simulink model "Simulator"  (R2016a)
settings: Solver=VariableStepAuto  StartTime=0.0  StopTime=10.0  RelTol=1e-6
undefined symbols (not defined in the file): eta_0, I_g, m, M_A, M_RB, nu_0, r_bg
libraries: SimulatorLibrary x5
settings Model: Creator=MortenFyhn  LastModifiedBy=vegard
settings DataIOCC: LimitDataPoints=on
settings DebuggingCC: AllowSymbolicDim=off
settings ModelReferenceCC: PropagateSignalLabelsOutOfModel=off
settings GRTTargetCC: GeneratePreprocessorConditionals=Use local settings

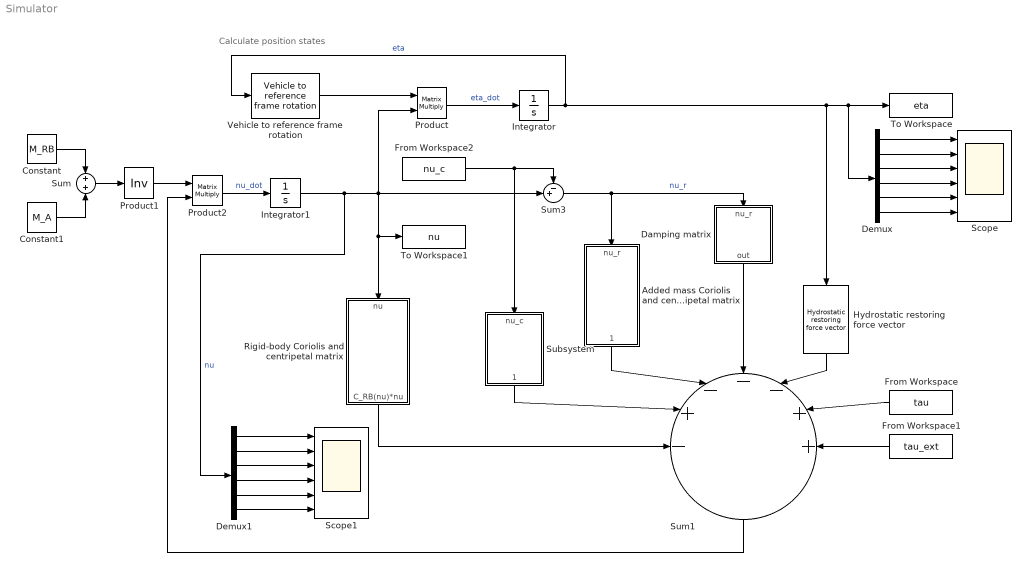
== system Simulator ==
  note: Calculate position states
  Added mass Coriolis and centripetal matrix : Subsystem
  Constant : Constant  Value=M_RB
  Constant1 : Constant  Value=M_A
  Damping matrix : Subsystem
  Demux : Demux  Outputs=6
  Demux1 : Demux  Outputs=6
  From Workspace : FromWorkspace  VariableName=tau  SampleTime=0
  From Workspace1 : FromWorkspace  VariableName=tau_ext  SampleTime=0
  From Workspace2 : FromWorkspace  VariableName=nu_c  SampleTime=0
  Hydrostatic restoring force vector : SimulatorLibrary/Hydrostatic restoring force vector
  Integrator : Integrator  InitialCondition=eta_0
  Integrator1 : Integrator  InitialCondition=nu_0
  Product : Product  Multiplication=Matrix(*)
  Product1 : Product  Inputs=/  Multiplication=Matrix(*)
  Product2 : Product  Multiplication=Matrix(*)
  Rigid-body Coriolis and centripetal matrix : Subsystem
  Scope : Scope  NumInputPorts=6
  Scope1 : Scope  NumInputPorts=6
  Subsystem : Subsystem
  Sum : Sum  Inputs=+|+
  Sum1 : Sum  Inputs=-+---++
  Sum3 : Sum  Inputs=-+|
  To Workspace : ToWorkspace  VariableName=eta  SaveFormat=Timeseries  SampleTime=-1
  To Workspace1 : ToWorkspace  VariableName=nu  SaveFormat=Timeseries  SampleTime=-1
  Vehicle to reference frame rotation : SimulatorLibrary/Vehicle to reference frame rotation
  wires:
  Vehicle to reference frame rotation/1 -> Product/1
  Product/1 -> Integrator/1  "eta_dot"
  Integrator/1 -> Vehicle to reference frame rotation/1, Demux/1, To Workspace/1, Hydrostatic restoring force vector/1  "eta"
  Constant1/1 -> Sum/2
  Constant/1 -> Sum/1
  Sum/1 -> Product1/1
  Product1/1 -> Product2/1
  Product2/1 -> Integrator1/1  "nu_dot"
  Integrator1/1 -> Demux1/1, To Workspace1/1, Rigid-body Coriolis and centripetal matrix/1(nu), Sum3/2, Product/2  "nu"
  Sum3/1 -> Added mass Coriolis and centripetal matrix/1(nu_r), Damping matrix/1(nu_r)  "nu_r"
  Sum1/1 -> Product2/2
  Hydrostatic restoring force vector/1 -> Sum1/5
  From Workspace/1 -> Sum1/6
  From Workspace1/1 -> Sum1/7
  Rigid-body Coriolis and centripetal matrix/1(C_RB(nu)*nu) -> Sum1/1
  Subsystem/1(M_A nu_c_dot) -> Sum1/2
  Added mass Coriolis and centripetal matrix/1(C_A(nu_r) nu_r) -> Sum1/3
  Damping matrix/1(out) -> Sum1/4
  From Workspace2/1 -> Subsystem/1(nu_c), Sum3/1
  Demux/6 -> Scope/6
  Demux/5 -> Scope/5
  Demux/4 -> Scope/4
  Demux/3 -> Scope/3
  Demux/2 -> Scope/2
  Demux/1 -> Scope/1
  Demux1/6 -> Scope1/6
  Demux1/5 -> Scope1/5
  Demux1/4 -> Scope1/4
  Demux1/3 -> Scope1/3
  Demux1/2 -> Scope1/2
  Demux1/1 -> Scope1/1

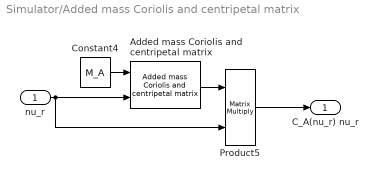
== system Simulator/Added mass Coriolis and centripetal matrix ==
  nu_r : Inport
  Added mass Coriolis and centripetal matrix : SimulatorLibrary/Added mass Coriolis and centripetal matrix
  Constant4 : Constant  Value=M_A
  Product5 : Product  Multiplication=Matrix(*)
  C_A(nu_r) nu_r : Outport
  wires:
  Constant4/1 -> Added mass Coriolis and centripetal matrix/1
  Added mass Coriolis and centripetal matrix/1 -> Product5/1
  nu_r/1 -> Product5/2, Added mass Coriolis and centripetal matrix/2
  Product5/1 -> C_A(nu_r) nu_r/1

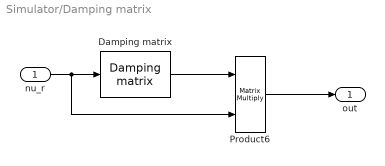
== system Simulator/Damping matrix ==
  nu_r : Inport
  Damping matrix : SimulatorLibrary/Damping matrix
  Product6 : Product  Multiplication=Matrix(*)
  out : Outport
  wires:
  Damping matrix/1 -> Product6/1
  nu_r/1 -> Product6/2, Damping matrix/1
  Product6/1 -> out/1

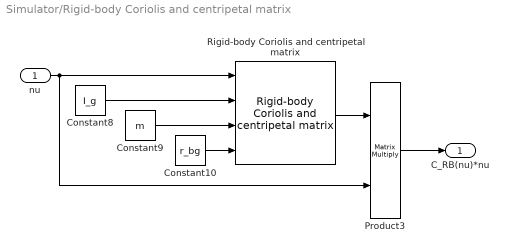
== system Simulator/Rigid-body Coriolis and centripetal matrix ==
  nu : Inport
  Constant10 : Constant  Value=r_bg
  Constant8 : Constant  Value=I_g
  Constant9 : Constant  Value=m
  Product3 : Product  Multiplication=Matrix(*)
  Rigid-body Coriolis and centripetal matrix : SimulatorLibrary/Rigid-body Coriolis and centripetal matrix
  C_RB(nu)*nu : Outport
  wires:
  Constant10/1 -> Rigid-body Coriolis and centripetal matrix/4
  Constant8/1 -> Rigid-body Coriolis and centripetal matrix/2
  Rigid-body Coriolis and centripetal matrix/1 -> Product3/1
  Constant9/1 -> Rigid-body Coriolis and centripetal matrix/3
  Product3/1 -> C_RB(nu)*nu/1
  nu/1 -> Product3/2, Rigid-body Coriolis and centripetal matrix/1

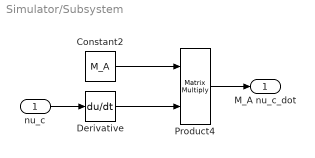
== system Simulator/Subsystem ==
  nu_c : Inport
  Constant2 : Constant  Value=M_A
  Derivative : Derivative
  Product4 : Product  Multiplication=Matrix(*)
  M_A nu_c_dot : Outport
  wires:
  Constant2/1 -> Product4/1
  Derivative/1 -> Product4/2
  Product4/1 -> M_A nu_c_dot/1
  nu_c/1 -> Derivative/1
